simulink model "MLimited"  (R2018b)
settings: Solver=FixedStepAuto  StartTime=0.0  StopTime=10.0  RelTol=1e-3
settings Model: DataDictionary=Master_Dictionary.sldd  Creator=torni  LastModifiedBy=oxbro
settings RTWCC: SystemTargetFile=irt.tlc  TemplateMakefile=irt_default_tmf  Description=INTECRIO Real-Time Target
settings STFCustomTargetCC: TargetLangStandard=C99 (ISO)  CombineOutputUpdateFcns=on  MatFileLogging=on  SystemTargetFile=irt.tlc
settings GRTTargetCC: ParMdlRefBuildCompliant=off  CompOptLevelCompliant=off  ConcurrentExecutionCompliant=off  CPPClassGenCompliant=off  UseToolchainInfoCompliant=off

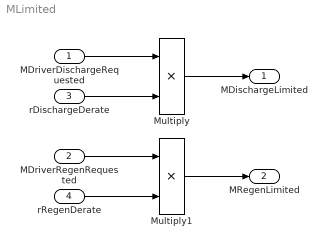
== system MLimited ==
  MDriverDischargeRequested : Inport  OutDataTypeStr=double
  MDriverRegenRequested : Inport  Port=2  OutDataTypeStr=double
  rDischargeDerate : Inport  Port=3  OutDataTypeStr=double
  rRegenDerate : Inport  Port=4  OutDataTypeStr=double
  Multiply : Product
  Multiply1 : Product
  MDischargeLimited : Outport  OutDataTypeStr=double
  MRegenLimited : Outport  Port=2  OutDataTypeStr=double
  wires:
  MDriverDischargeRequested/1 -> Multiply/1
  rDischargeDerate/1 -> Multiply/2
  MDriverRegenRequested/1 -> Multiply1/1
  rRegenDerate/1 -> Multiply1/2
  Multiply/1 -> MDischargeLimited/1
  Multiply1/1 -> MRegenLimited/1
